simulink model "SVPWM_2level"  (R2024a)
settings: Solver=ode3  StartTime=0.0  StopTime=0.1  RelTol=1e-3
InitFcn:
  | fs=1550
  | Ts=1/1550
libraries: spsVoltageMeasurementLib x9, spsIGBTDiodeLib x6, spsCurrentMeasurementLib x3, spsSeriesRLCBranchLib x3, spsabctoAlphaBetaZeroLib x2, simulink_extras x1, simulink x1, spsDCVoltageSourceLib x1, spsGroundLib x1, spspowerguiLib x1
settings Model: Creator=aayus  LastModifiedBy=bpven
settings DataIOCC: SaveFormat=StructureWithTime  SaveTime=off  ReturnWorkspaceOutputs=off
settings RTWCC: GPUComputeCapability=3.5

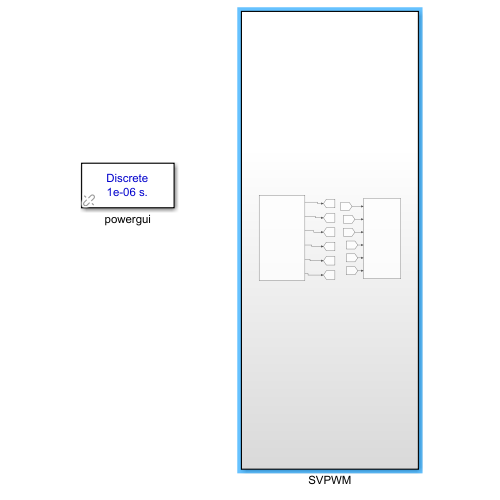
[thumbnail: Simulink's stored preview of the top-level diagram]
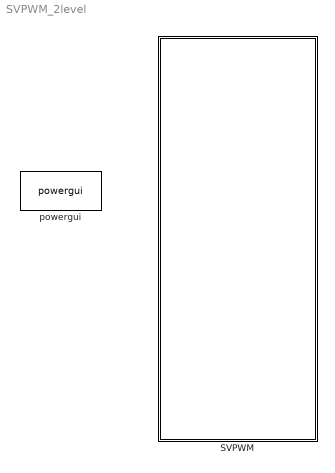
== system SVPWM_2level ==
  SVPWM : Subsystem
  powergui : spspowerguiLib/powergui  Priority=1  SimulationMode=Discrete  SampleTime=1e-6  frequency=60  Iterations=50  frequencyindice=0  Pbase=100e6  ErrMax=1e-4  UnitsV=kV  UnitsW=MW  buscounter=0  FunctionMessages=off  echomessages=off  EnableUseOfTLC=off  CurrentSourceSwitches=off  DisableSnubberDevices=off  DisableRonSwitches=off  DisableVfSwitches=off  DisplayEquations=off  AutomaticDiscreteSolvers=off  SolverType=Tustin/Backward Euler (TBE)  Interpol=off  ExternalGateDelay=off  methode=off  Ts=100  x0status=blocks  SPID=on  SwTol=0  HookPort=off  NonlinearTolerance=1e-4  nMaxIteration=100  ContinueOnMaxIteration=off  RestoreLinks=warning  ResistiveCurrentMeasurement=off  Frange=[0:2:500]  Ylog=off  Xlog=on  ShowGrid=off  save=off  variable=ZData  structure=0  ZoomFFT=off  StartTime=0.0  cycles=1  DisplayStyle=1  fundamental=60  FreqAxis=off  MaxFrequency=1000  frequencyindicesteady=1  RmsSteady=1  display=off

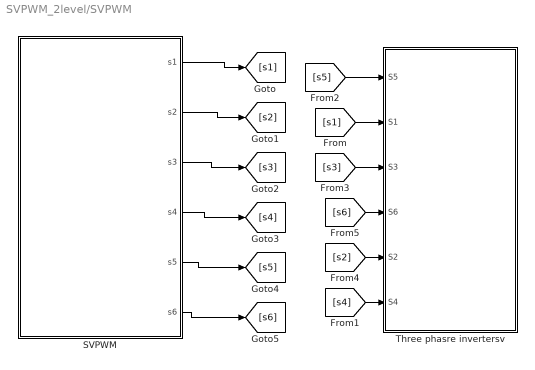
== system SVPWM_2level/SVPWM ==
  SVPWM : Subsystem
  Three phasre invertersv : Subsystem
  wires:
  [s1] -> Three phasre invertersv/2(S1)
  [s5] -> Three phasre invertersv/1(S5)
  [s3] -> Three phasre invertersv/3(S3)
  SVPWM/6(s6) -> [s6]
  SVPWM/5(s5) -> [s5]
  [s6] -> Three phasre invertersv/4(S6)
  SVPWM/1(s1) -> [s1]
  SVPWM/2(s2) -> [s2]
  SVPWM/4(s4) -> [s4]
  SVPWM/3(s3) -> [s3]
  [s2] -> Three phasre invertersv/5(S2)
  [s4] -> Three phasre invertersv/6(S4)

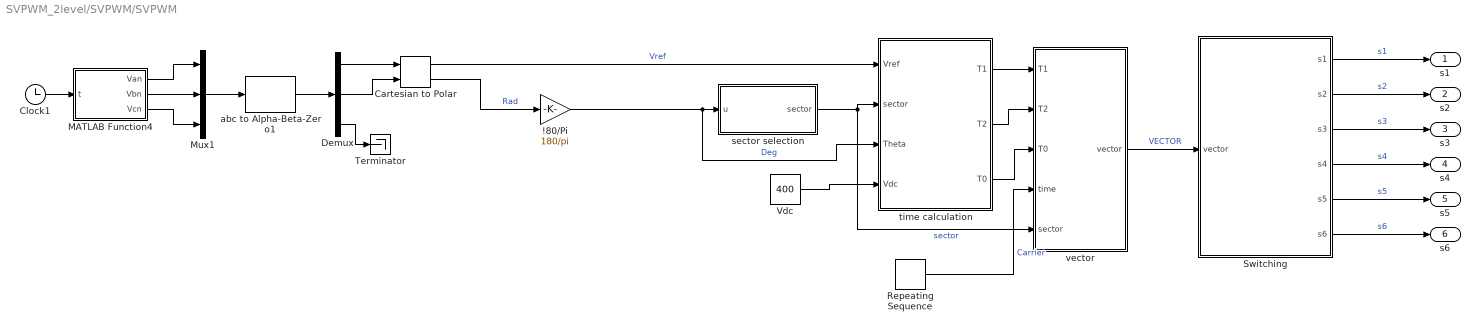
== system SVPWM_2level/SVPWM/SVPWM ==
  !80/Pi : Gain  Gain=180/pi
  Cartesian to Polar : simulink_extras/Transformations/Cartesian to Polar
  Clock1 : Clock
  Demux : Demux  Outputs=3
  MATLAB Function4 : MATLAB Function  TreatAsAtomicUnit=on
  Mux1 : Mux  Inputs=3
  Repeating Sequence : simulink/Sources/Repeating Sequence  rep_seq_t=[0 0.5 1]*(1/1550)  rep_seq_y=[0 0.5 1]*(1/1550)
  Switching : MATLAB Function  TreatAsAtomicUnit=on
  Terminator : Terminator
  Vdc : Constant  Value=400
  abc to Alpha-Beta-Zero1 : spsabctoAlphaBetaZeroLib/abc to Alpha-Beta-Zero
  sector selection : MATLAB Function  TreatAsAtomicUnit=on
  time calculation : MATLAB Function  TreatAsAtomicUnit=on
  vector : MATLAB Function  TreatAsAtomicUnit=on
  s1 : Outport
  s2 : Outport  Port=2
  s3 : Outport  Port=3
  s4 : Outport  Port=4
  s5 : Outport  Port=5
  s6 : Outport  Port=6
  wires:
  Clock1/1 -> MATLAB Function4/1(t)
  sector selection/1(sector) -> vector/5(sector), time calculation/2(sector)  "sector"
  Switching/2(s2) -> s2/1  "s2"
  MATLAB Function4/2(Vbn) -> Mux1/2
  !80/Pi/1 -> time calculation/3(Theta), sector selection/1(u)  "Deg"
  MATLAB Function4/3(Vcn) -> Mux1/3
  Switching/5(s5) -> s5/1  "s5"
  Demux/2 -> Cartesian to Polar/2
  abc to Alpha-Beta-Zero1/1 -> Demux/1
  vector/1(vector) -> Switching/1(vector)  "VECTOR"
  Mux1/1 -> abc to Alpha-Beta-Zero1/1
  Demux/3 -> Terminator/1
  Vdc/1 -> time calculation/4(Vdc)
  Switching/1(s1) -> s1/1  "s1"
  Demux/1 -> Cartesian to Polar/1
  Repeating Sequence/1 -> vector/4(time)  "Carrier"
  MATLAB Function4/1(Van) -> Mux1/1
  time calculation/3(T0) -> vector/3(T0)
  Cartesian to Polar/1 -> time calculation/1(Vref)  "Vref"
  time calculation/1(T1) -> vector/1(T1)
  Cartesian to Polar/2 -> !80/Pi/1  "Rad"
  time calculation/2(T2) -> vector/2(T2)
  Switching/3(s3) -> s3/1  "s3"
  Switching/6(s6) -> s6/1  "s6"
  Switching/4(s4) -> s4/1  "s4"

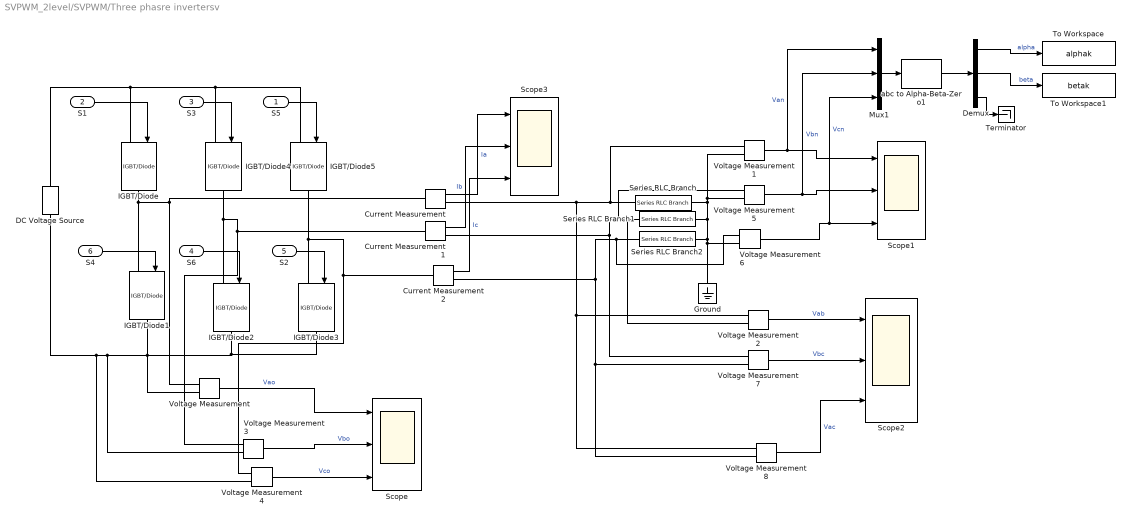
== system SVPWM_2level/SVPWM/Three phasre invertersv ==
  S5 : Inport
  S1 : Inport  Port=2
  S3 : Inport  Port=3
  S6 : Inport  Port=4
  S2 : Inport  Port=5
  S4 : Inport  Port=6
  Current Measurement : spsCurrentMeasurementLib/Current Measurement  PhasorSimulation=off  OutputType=Complex  PSBequivalent=0
  Current Measurement1 : spsCurrentMeasurementLib/Current Measurement  PhasorSimulation=off  OutputType=Complex  PSBequivalent=0
  Current Measurement2 : spsCurrentMeasurementLib/Current Measurement  PhasorSimulation=off  OutputType=Complex  PSBequivalent=0
  DC Voltage Source : spsDCVoltageSourceLib/DC Voltage Source  Amplitude=400  Measurements=None
  Demux : Demux  Outputs=3
  Ground : spsGroundLib/Ground  LConnTagsString=a
  IGBT/Diode{,1..5} (6 alike) : spsIGBTDiodeLib/IGBT//Diode  Ron=1e-3  Rs=1e5  Cs=inf  Measurements=off
  Mux1 : Mux  Inputs=3
  Scope{,1..3} (4 alike) : Scope  NumInputPorts=3
  Series RLC Branch : spsSeriesRLCBranchLib/Series RLC Branch  LConnTagsString=__new0  RConnTagsString=__new0  BranchType=L  Resistance=1  Inductance=1e-3  SetiL0=off  InitialCurrent=0  Capacitance=1e-6  Setx0=off  InitialVoltage=0  Measurements=Branch voltage and current
  Series RLC Branch1 : spsSeriesRLCBranchLib/Series RLC Branch  LConnTagsString=__new0  RConnTagsString=__new0  BranchType=L  Resistance=1  Inductance=1e-3  SetiL0=off  InitialCurrent=0  Capacitance=1e-6  Setx0=off  InitialVoltage=0  Measurements=Branch voltage and current
  Series RLC Branch2 : spsSeriesRLCBranchLib/Series RLC Branch  LConnTagsString=__new0  RConnTagsString=__new0  BranchType=L  Resistance=1  Inductance=1e-3  SetiL0=off  InitialCurrent=0  Capacitance=1e-6  Setx0=off  InitialVoltage=0  Measurements=Branch voltage and current
  Terminator : Terminator
  To Workspace : ToWorkspace  VariableName=alphak  SampleTime=-1
      settings: Save2DSignal=2-D array (concatenate along first dimension)
  To Workspace1 : ToWorkspace  VariableName=betak  SampleTime=-1
      settings: Save2DSignal=2-D array (concatenate along first dimension)
  Voltage Measurement{,1..8} (9 alike) : spsVoltageMeasurementLib/Voltage Measurement  PhasorSimulation=off  OutputType=Complex  PSBequivalent=0
  abc to Alpha-Beta-Zero1 : spsabctoAlphaBetaZeroLib/abc to Alpha-Beta-Zero
  wires:
  Current Measurement/1 -> Scope3/1  "Ia"
  Demux/1 -> To Workspace/1  "alpha"
  Demux/3 -> Terminator/1
  Demux/2 -> To Workspace1/1  "beta"
  abc to Alpha-Beta-Zero1/1 -> Demux/1
  S5/1 -> IGBT/Diode5/1
  Mux1/1 -> abc to Alpha-Beta-Zero1/1
  S4/1 -> IGBT/Diode1/1
  Current Measurement2/1 -> Scope3/3  "Ic"
  Current Measurement1/1 -> Scope3/2  "Ib"
  Voltage Measurement8/1 -> Scope2/3  "Vac"
  Voltage Measurement5/1 -> Scope1/2, Mux1/2  "Vbn"
  Voltage Measurement/1 -> Scope/1  "Vao"
  Voltage Measurement7/1 -> Scope2/2  "Vbc"
  Voltage Measurement3/1 -> Scope/2  "Vbo"
  S1/1 -> IGBT/Diode/1
  S3/1 -> IGBT/Diode4/1
  Voltage Measurement2/1 -> Scope2/1  "Vab"
  S6/1 -> IGBT/Diode2/1
  Voltage Measurement1/1 -> Mux1/1, Scope1/1  "Van"
  S2/1 -> IGBT/Diode3/1
  Voltage Measurement6/1 -> Mux1/3, Scope1/3  "Vcn"
  Voltage Measurement4/1 -> Scope/3  "Vco"
  connections:
  Voltage Measurement7/LConn2 -- Voltage Measurement8/LConn2 -- Voltage Measurement6/LConn1 -- Series RLC Branch2/LConn1 -- Current Measurement2/RConn1
  IGBT/Diode4/LConn1 -- IGBT/Diode5/LConn1 -- DC Voltage Source/RConn1 -- IGBT/Diode/LConn1
  Voltage Measurement3/LConn1 -- IGBT/Diode4/RConn1 -- IGBT/Diode2/LConn1 -- Current Measurement1/LConn1
  Voltage Measurement6/LConn2 -- Voltage Measurement5/LConn2 -- Voltage Measurement1/LConn2 -- Series RLC Branch/RConn1 -- Series RLC Branch1/RConn1 -- Series RLC Branch2/RConn1 -- Ground/LConn1
  Voltage Measurement7/LConn1 -- Current Measurement1/RConn1 -- Voltage Measurement2/LConn2 -- Series RLC Branch1/LConn1 -- Voltage Measurement5/LConn1
  Voltage Measurement2/LConn1 -- Voltage Measurement1/LConn1 -- Series RLC Branch/LConn1 -- Current Measurement/RConn1 -- Voltage Measurement8/LConn1
  Current Measurement/LConn1 -- Voltage Measurement/LConn1 -- IGBT/Diode/RConn1 -- IGBT/Diode1/LConn1
  IGBT/Diode1/RConn1 -- Voltage Measurement3/LConn2 -- Voltage Measurement4/LConn2 -- DC Voltage Source/LConn1 -- Voltage Measurement/LConn2 -- IGBT/Diode3/RConn1 -- IGBT/Diode2/RConn1
  Current Measurement2/LConn1 -- Voltage Measurement4/LConn1 -- IGBT/Diode5/RConn1 -- IGBT/Diode3/LConn1

== matlab function SVPWM_2level/SVPWM/SVPWM/MATLAB Function4 ==
  data: t input; Van output; Vbn output; Vcn output
function [Van,Vbn,Vcn] = fcn(t)

w=2*pi*50
theta1=2*pi/3
theta2=4*pi/3
Van=230*sin(w*t)
Vbn=230*sin(w*t-theta1)
Vcn=230*sin(w*t-theta2)
end

== matlab function SVPWM_2level/SVPWM/SVPWM/Switching ==
  data: vector input; s1 output; s2 output; s3 output; s4 output; s5 output; s6 output
function [s1,s2,s3,s4,s5,s6] = fcn(vector)
    s1=0;
    s2=0;
    s3=0;      
    s4=0;
    s5=0;
    s6=0;
if(vector==1)
    s1=1;
    s2=1;
    s3=0;      %100
    s4=0;
    s5=0;
    s6=1;
elseif(vector==2)
    s1=1;
    s2=1;
    s3=1;
    s4=0;      %110
    s5=0;
    s6=0;
elseif(vector==3)
    s1=0;
    s2=1;
    s3=1;
    s4=1;      %010
    s5=0;
    s6=0;
elseif(vector==4)
    s1=0;
    s2=0;
    s3=1;
    s4=1;    %011
    s5=1;
    s6=0;
elseif(vector==5)
    s1=0;
    s2=0;
    s3=0;
    s4=1;    %001
    s5=1;
    s6=1;
elseif(vector==6)
    s1=1;
    s2=0;
    s3=0;        %101    
    s4=0;
    s5=1;
    s6=1;
elseif(vector==7)
    s1=1;
    s2=0;
    s3=1;
    s4=0;        %111
    s5=1;
    s6=0;
elseif(vector==8)
    s1=0;
    s2=1;
    s3=0;        %000
    s4=1;
    s5=0;
    s6=1;
end

Switiching = [s1,s2,s3,s4,s5,s6];
end

== matlab function SVPWM_2level/SVPWM/SVPWM/sector selection ==
  data: u input; sector output
function sector = fcn(u)

angle = u(1);

if(60>=angle && angle>0)
    sector=1;
elseif(120>=angle && angle>60)  
    sector=2;
elseif(180>=angle && angle>120)
    sector=3;
elseif(-120>=angle && angle>-180)
    sector=4;
elseif(-60>=angle && angle>-120)
    sector=5;
else
    sector=6;
 
end
end

== matlab function SVPWM_2level/SVPWM/SVPWM/time calculation ==
  data: Vref input; T1 output; sector input; Theta input; Vdc input; T2 output; T0 output
function [T1,T2,T0] = fcn(Vref,sector,Theta,Vdc)

ma=sqrt(3)*Vref/Vdc ;
Ts= 1/1550;
Theta_rad=Theta*(pi/180);
Adv_Theta_rad= Theta_rad-(sector-1)*(pi/3);
T1=Ts*ma*sin(pi/3 - Adv_Theta_rad);
T2=Ts*ma*sin(Adv_Theta_rad);
T0=Ts-T1-T2;
end

== matlab function SVPWM_2level/SVPWM/SVPWM/vector ==
  data: T1 input; vector output; T2 input; T0 input; time input; sector input
function vector = fcn(T1,T2,T0,time,sector)
vector=8;
% for sector 1 3 5

tt1=T0/4 ;
tt2=tt1+T1/2;
tt3=tt2+T2/2;
tt4=tt3+T0/2;
tt5=tt4+T2/2;
tt6=tt5+T1/2;
%tt7=tt6+T0/4;

% for sector 2 4 6
t1=T0/4;
t2=t1+T2/2;
t3=t2+T1/2;
t4=t3+T0/2;
t5=t4+T1/2;
t6=t5+T2/2;
%t7=t6+T0/4;


if(sector==1)

    if(time>0 && time <= tt1)
        vector=8;
    elseif(time>tt1 && time <= tt2)
        vector=1;
    elseif(time>tt2 && time <= tt3)
        vector=2;
    elseif(time>tt3 && time <= tt4)
        vector=7;
    elseif(time>tt4 && time <= tt5)
        vector=2;
    elseif(time>tt5 && time <= tt6)
        vector=1;
    else
        vector=8;
    end
    
    
elseif(sector==3)

    if(time>0 && time <= tt1)
        vector=8;
    elseif(time>tt1 && time <= tt2)
        vector=3;
    elseif(time>tt2 && time <= tt3)
        vector=4;
    elseif(time>tt3 && time <= tt4)
        vector=7;
    elseif(time>tt4 && time <= tt5)
        vector=4;
    elseif(time>tt5 && time <= tt6)
        vector=3;
    else
        vector=8;
    end

elseif(sector==5)

    if(time>0 && time <= tt1)
        vector=8;
    elseif(time>tt1 && time <= tt2)
        vector=5;
    elseif(time>tt2 && time <= tt3)
        vector=6;
    elseif(time>tt3 && time <= tt4)
        vector=7;
    elseif(time>tt4 && time <= tt5)
        vector=6;
    elseif(time>tt5 && time <= tt6)
        vector=5;
    else
        vector=8;
    end
elseif(sector==2)
    if(time>0 && time <= t1)
        vector=8;
    elseif(time>t1 && time <= t2)
        vector=3;
    elseif(time>t2 && time <= t3)
        vector=2;
    elseif(time>t3 && time <= t4)
        vector=7;
    elseif(time>t4 && time <= t5)
        vector=2;
    elseif(time>t5 && time <= t6)
        vector=3;
    else
        vector=8;
    end

elseif(sector==4)

    if(time>0 && time <= t1)
        vector=8;
    elseif(time>t1 && time <= t2)
        vector=5;
    elseif(time>t2 && time <= t3)
        vector=4;
    elseif(time>t3 && time <= t4)
        vector=7;
    elseif(time>t4 && time <= t5)
        vector=4;
    elseif(time>t5 && time <= t6)
        vector=5;
    else
        vector=8;
    end

elseif(sector==6)

    if(time>0 && time <= t1)
        vector=8;
    elseif(time>t1 && time <= t2)
        vector=1;
    elseif(time>t2 && time <= t3)
        vector=6;
    elseif(time>t3 && time <= t4)
        vector=7;
    elseif(time>t4 && time <= t5)
        vector=6;
    elseif(time>t5 && time <= t6)
        vector=1;
    else
        vector=8;
    end
end
end
